simulink model "submarino"  (R2021a)
settings: Solver=VariableStepAuto  StartTime=0.0  StopTime=10.0  RelTol=1e-3
settings Model: Creator=OSCAR  LastModifiedBy=OSCAR

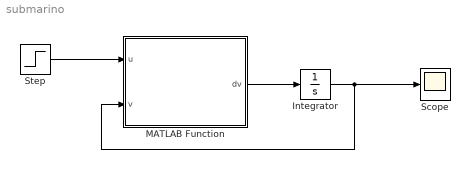
== system submarino ==
  Integrator : Integrator
  MATLAB Function : MATLAB Function  TreatAsAtomicUnit=on
  Scope : Scope
  Step : Step  Time=0  SampleTime=0
  wires:
  MATLAB Function/1(dv) -> Integrator/1
  Integrator/1 -> Scope/1, MATLAB Function/2(v)
  Step/1 -> MATLAB Function/1(u)

== matlab function submarino/MATLAB Function ==
  data: u input; dv output; v input
function dv = submarino(u,v)

dv = u - abs(v)*v;
